simulink subsystem "loggingsub"  (R2020b)
settings: Solver=VariableStepAuto  StartTime=0.0  StopTime=10.0  RelTol=1e-3
settings Model: Creator=MSI PC  LastModifiedBy=MSI PC

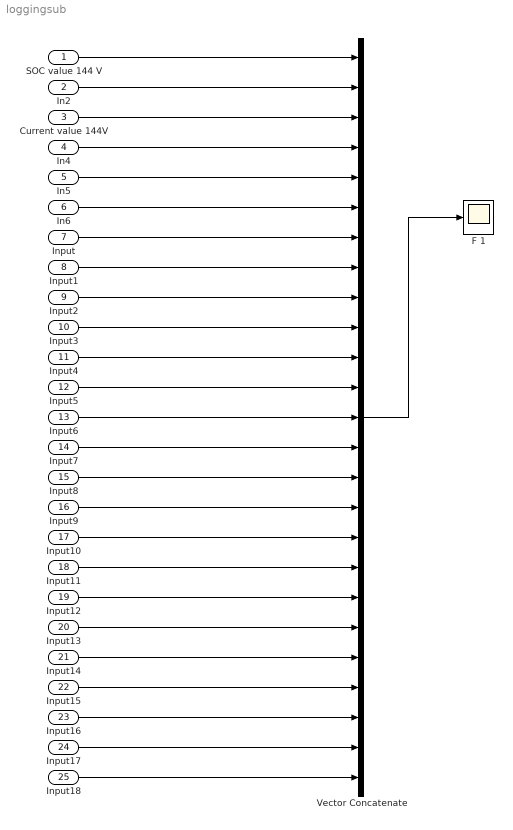
== system loggingsub ==
  SOC value 144 V : Inport
  In2 : Inport  Port=2
  Current value 144V : Inport  Port=3
  In4 : Inport  Port=4
  In5 : Inport  Port=5
  In6 : Inport  Port=6
  Input : Inport  Port=7
  Input1 : Inport  Port=8
  Input2 : Inport  Port=9
  Input3 : Inport  Port=10
  Input4 : Inport  Port=11
  Input5 : Inport  Port=12
  Input6 : Inport  Port=13
  Input7 : Inport  Port=14
  Input8 : Inport  Port=15
  Input9 : Inport  Port=16
  Input10 : Inport  Port=17
  Input11 : Inport  Port=18
  Input12 : Inport  Port=19
  Input13 : Inport  Port=20
  Input14 : Inport  Port=21
  Input15 : Inport  Port=22
  Input16 : Inport  Port=23
  Input17 : Inport  Port=24
  Input18 : Inport  Port=25
  F 1 : Scope
  Vector Concatenate : Concatenate  NumInputs=25
  wires:
  Vector Concatenate/1 -> F 1/1
  In5/1 -> Vector Concatenate/5
  In2/1 -> Vector Concatenate/2
  In4/1 -> Vector Concatenate/4
  Current value 144V/1 -> Vector Concatenate/3
  In6/1 -> Vector Concatenate/6
  SOC value 144 V/1 -> Vector Concatenate/1
  Input/1 -> Vector Concatenate/7
  Input1/1 -> Vector Concatenate/8
  Input2/1 -> Vector Concatenate/9
  Input3/1 -> Vector Concatenate/10
  Input4/1 -> Vector Concatenate/11
  Input5/1 -> Vector Concatenate/12
  Input6/1 -> Vector Concatenate/13
  Input7/1 -> Vector Concatenate/14
  Input8/1 -> Vector Concatenate/15
  Input9/1 -> Vector Concatenate/16
  Input10/1 -> Vector Concatenate/17
  Input18/1 -> Vector Concatenate/25
  Input17/1 -> Vector Concatenate/24
  Input16/1 -> Vector Concatenate/23
  Input15/1 -> Vector Concatenate/22
  Input14/1 -> Vector Concatenate/21
  Input13/1 -> Vector Concatenate/20
  Input12/1 -> Vector Concatenate/19
  Input11/1 -> Vector Concatenate/18
